simulink model "MultiVehicleModel"  (R2014a)
settings: Solver=ode1  StartTime=0.0  StopTime=inf  FixedStep=simPars.SampleTime  RelTol=1e-3
undefined symbols (not defined in the file or in its folder): DiscIntNeverNeededParam, Earth, Env, eul_0, FWFleet, GVFleet, m, RCFleet, s, WGS84
undefined symbols (not defined in the file): simPars
libraries: simulink x26, aerolibtransform2 x7, instrumentlib x6, Actuator_Lib x5, aerolib6dofsys x4, etargetslib x3, aerolibasang x3, aerolibconvert2 x2, aerolibutil x1, aerolibatmos2 x1, aerolibobsolete x1, aerolibgravity2 x1
(part 1 of 4)
settings Model: SimulationMode=accelerator  Creator=Paul Freeman  LastModifiedBy=Justyna
settings DataIOCC: LimitDataPoints=off  SignalLoggingSaveFormat=ModelDataLogs  SaveOutput=off  SignalLogging=off
settings OptimizationCC: ExpressionDepthLimit=2147483647  EfficientMapNaN2IntZero=off
settings DebuggingCC: UnderspecifiedInitializationDetection=Classic  MultiTaskDSMMsg=warning  MultiTaskCondExecSysMsg=none  FcnCallInpInsideContextMsg=UseLocalSettings  StateNameClashWarn=warning
settings HardwareCC: ProdLargestAtomicInteger=Long  ProdLargestAtomicFloat=Double  ProdIntDivRoundTo=Zero  ProdEndianess=BigEndian  ProdHWDeviceType=Freescale->32-bit PowerPC  TargetIntDivRoundTo=Zero  TargetEndianess=LittleEndian  TargetHWDeviceType=MATLAB Host  ProdEqTarget=off
settings SFSimCC: SimParseCustomCode=off
settings CodeAppCC: MaxIdLength=128
settings GRTTargetCC: CombineOutputUpdateFcns=off  GRTInterface=on

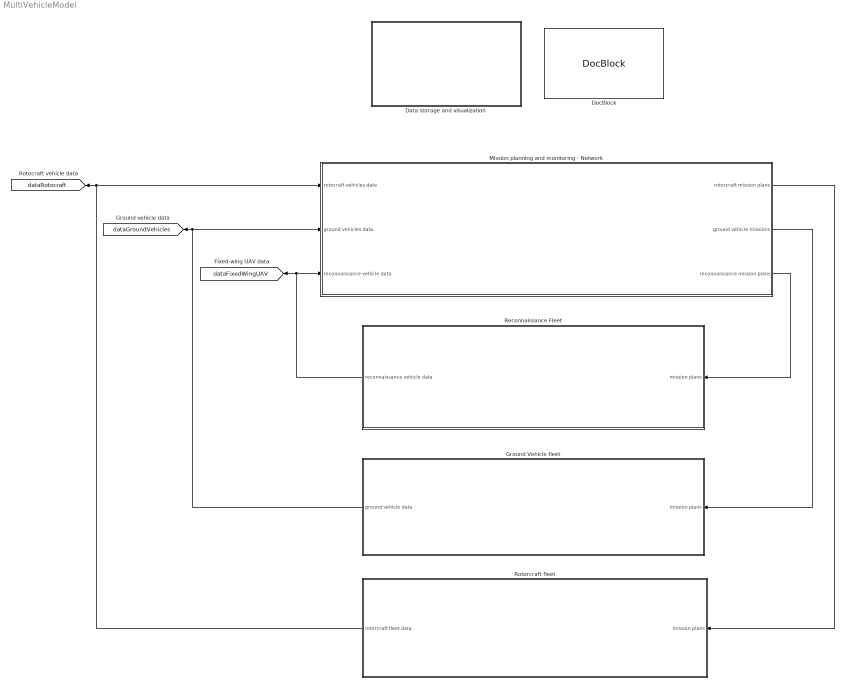
== system MultiVehicleModel ==
  Data storage and visualization : Subsystem
  DocBlock : simulink/Model-Wide Utilities/DocBlock  DocumentType=Text
      content=|
      | Type your documentation here
  Ground Vehicle fleet : Subsystem
  Mission planning and monitoring - Network : Subsystem  RequirementInfo={'other' 'specs1.mn' '@1.1.' 'true' 'specs' '' } %GIDa_c3d0c7d9_1841_4ce2_80a1_9c96a4f97ba6
  Reconnaissance Fleet : Subsystem
  Rotorcraft fleet : Subsystem
  tag scope: dataFixedWingUAV=global, dataGroundVehicles=global, dataRotocraft=global
  wires:
  Reconnaissance Fleet/1(reconnaissance vehicle data) -> [dataFixedWingUAV], Mission planning and monitoring - Network/3(reconnaissance vehicle data)
  Mission planning and monitoring - Network/3(reconnaissance mission plans) -> Reconnaissance Fleet/1(mission plans)
  Ground Vehicle fleet/1(ground vehicle data) -> [dataGroundVehicles], Mission planning and monitoring - Network/2(ground vehicles data)
  Rotorcraft fleet/1(rotorcraft fleet data) -> [dataRotocraft], Mission planning and monitoring - Network/1(rotocraft vehicles data)
  Mission planning and monitoring - Network/2(ground vehicle missions) -> Ground Vehicle fleet/1("mission plans ")
  Mission planning and monitoring - Network/1(rotorcraft mission plans) -> Rotorcraft fleet/1(mission plans)

== system MultiVehicleModel/Data storage and visualization ==
  To Workspace : ToWorkspace  VariableName=dataFixedWingUAV  SaveFormat=Structure With Time  SampleTime=-1
  To Workspace1 : ToWorkspace  VariableName=dataGroundVehicles  SaveFormat=Structure With Time  SampleTime=-1
  To Workspace2 : ToWorkspace  VariableName=dataRotorcraft  SaveFormat=Structure With Time  SampleTime=-1
  wires:
  [dataRotocraft] -> To Workspace2/1
  [dataGroundVehicles] -> To Workspace1/1
  [dataFixedWingUAV] -> To Workspace/1

== system MultiVehicleModel/Ground Vehicle fleet ==
  "mission plans " : Inport
  Bus Selector : BusSelector  OutputSignals=Ground vehicle fleet waypoints,Ground vehicle fleet functions
  Initial North-East-Down position : Constant  Value=GVFleet.IC.posNED(1:2,:)  VectorParams1D=off
  Model of ground vehicle fleet : Subsystem  TreatAsAtomicUnit=on  mask{AC=FWFleet.AC, Env=Env, SampleTime=simPars.SampleTime}
      mask prompts: AC "Aircraft properties"; Env "Environmental parameters"; SampleTime "Sample time (sec)"
  data inertial coordinates for debug. : ToWorkspace  VariableName=dataGVInertial  SaveFormat=Structure With Time  SampleTime=-1
  ground vehicle data : Outport
  wires:
  Model of ground vehicle fleet/1(output data) -> ground vehicle data/1
  Bus Selector/1 -> Model of ground vehicle fleet/1(air controller data)  "<Ground vehicle fleet waypoints>"
  Bus Selector/2 -> Model of ground vehicle fleet/2(AC fcn)  "<Ground vehicle fleet functions>"
  "mission plans "/1 -> Bus Selector/1
  Initial North-East-Down position/1 -> Model of ground vehicle fleet/3(Initial conditions)
  Model of ground vehicle fleet/2(output data inertial) -> data inertial coordinates for debug./1

== system MultiVehicleModel/Mission planning and monitoring - Network ==
  rotocraft vehicles data : Inport
  ground vehicles data : Inport  Port=2
  reconnaissance vehicle data : Inport  Port=3
  "Mission Plan Generation for fixed wing UAV fleet Runs on the server / cloud " : Subsystem
  Mission Plan Generation for ground vehicle fleet Runs on the server / cloud : Subsystem
  Mission Plan Generation for rotorcraft fleet Runs on the server / cloud : Subsystem
  rotorcraft mission plans : Outport
  ground vehicle missions : Outport  Port=2
  reconnaissance mission plans : Outport  Port=3
  wires:
  "Mission Plan Generation for fixed wing UAV fleet Runs on the server / cloud "/1(vehicle mission plans) -> reconnaissance mission plans/1  "vehicle mission plans"
  reconnaissance vehicle data/1 -> "Mission Plan Generation for fixed wing UAV fleet Runs on the server / cloud "/1(reconnaissance vehicle data)
  Mission Plan Generation for rotorcraft fleet Runs on the server / cloud/1(vehicle mission plans) -> rotorcraft mission plans/1
  ground vehicles data/1 -> Mission Plan Generation for ground vehicle fleet Runs on the server / cloud/1(ground vehicle data)
  rotocraft vehicles data/1 -> Mission Plan Generation for rotorcraft fleet Runs on the server / cloud/1(rotorcraft vehicle data)
  Mission Plan Generation for ground vehicle fleet Runs on the server / cloud/1(vehicle mission plans) -> ground vehicle missions/1

== system MultiVehicleModel/Reconnaissance Fleet ==
  mission plans : Inport
  Bus Selector : BusSelector  OutputSignals=Fixed-wing UAV fleet waypoints,Fixed-wing UAV fleet functions
  Initial North-East-Down position : Constant  Value=FWFleet.IC.posNED  VectorParams1D=off
  Initial heading : Constant  Value=FWFleet.IC.heading  VectorParams1D=off
  Matrix Concatenate : Concatenate  Mode=Multidimensional array
  UMN - Uninhabited Aerial Vehicle Fleet : Subsystem  TreatAsAtomicUnit=on  mask{AC=FWFleet.AC, Env=Env, SampleTime=simPars.SampleTime}
      mask prompts: AC "Aircraft properties"; Env "Environmental parameters"; SampleTime "Sample time (sec)"
  reconnaissance vehicle data : Outport
  wires:
  UMN - Uninhabited Aerial Vehicle Fleet/1(output data) -> reconnaissance vehicle data/1
  Bus Selector/1 -> UMN - Uninhabited Aerial Vehicle Fleet/1(mission plan)  "<Fixed-wing UAV fleet waypoints>"
  Bus Selector/2 -> UMN - Uninhabited Aerial Vehicle Fleet/2(Function)  "<Fixed-wing UAV fleet functions>"
  mission plans/1 -> Bus Selector/1
  Initial North-East-Down position/1 -> Matrix Concatenate/1
  Initial heading/1 -> Matrix Concatenate/2
  Matrix Concatenate/1 -> UMN - Uninhabited Aerial Vehicle Fleet/3(A/C initial conditions)

== system MultiVehicleModel/Rotorcraft fleet ==
  mission plans : Inport
  Bus Selector : BusSelector  OutputSignals="AR fleet waypoints,AR fleet heading and time,AR  fleet functions"
  Initial North-East-Down position : Constant  Value=RCFleet.IC.posNED  VectorParams1D=off
  Initial heading : Constant  Value=RCFleet.IC.heading  VectorParams1D=off
  Matrix Concatenate : Concatenate  Mode=Multidimensional array
  Multiple Rotorcraft : Subsystem  TreatAsAtomicUnit=on  mask{RCFleet=RCFleet}
      mask prompts: RCFleet "Rotorcraft fleet data structure"
  data inertial coordinates for debug. : ToWorkspace  VariableName=dataRotocraft2  SaveFormat=Structure With Time  SampleTime=-1
  rotorcraft fleet data : Outport
  wires:
  Multiple Rotorcraft/1(fleet states) -> rotorcraft fleet data/1
  Bus Selector/1 -> Multiple Rotorcraft/1(waypoints)  "<AR fleet waypoints>"
  Bus Selector/3 -> Multiple Rotorcraft/3(fleet functions)  "<AR  fleet functions>"
  mission plans/1 -> Bus Selector/1
  Multiple Rotorcraft/2(fleet inertial) -> data inertial coordinates for debug./1
  Bus Selector/2 -> Multiple Rotorcraft/2(heading and time references)  "<AR fleet heading and time>"
  Initial North-East-Down position/1 -> Matrix Concatenate/1
  Initial heading/1 -> Matrix Concatenate/2
  Matrix Concatenate/1 -> Multiple Rotorcraft/4(initial conditions)

== system MultiVehicleModel/Ground Vehicle fleet/Model of ground vehicle fleet ==
  air controller data : Inport  Partition=on  PartitionDimension=3  PartitionWidth=1
  AC fcn : Inport  Port=2  Partition=on  PartitionDimension=1  PartitionWidth=1
  Initial conditions : Inport  Port=3  Partition=on  PartitionDimension=2  PartitionWidth=1
  Bus Creator : BusCreator  Inputs=2
  Bus Selector1 : BusSelector  OutputSignals=Pned (m),psi (rad)
  Demux : Demux  Outputs=3
  Guidance algorithm : Subsystem
  Iteration over the UAV fleet : ForEach  DisableCoverage=on  IndexMode=One-based
  Mux1 : Mux
  Navigation : Subsystem  Description=|
      | This model produces the followng navigation data for the UAV flight:
      |                                                                     
      | * Geodetic Latitude                                                 
      | * Geodetic Longitude                                                
      | * Geodetic Altitude                                                 
      | * Altitude above Mean Sea Level                                     
      | * Gravitational acceleration vector
  Very simple car model : Subsystem
  data to send : Subsystem
  output data : Outport  ConcatenationDimension=1
  output data inertial : Outport  Port=2  ConcatenationDimension=1
  wires:
  air controller data/1 -> Guidance algorithm/2(waypoint data)
  AC fcn/1 -> Guidance algorithm/3(AC fcn)
  Very simple car model/1(position) -> Bus Creator/1, Navigation/1(X_e [m])  "Pned (m)"
  Very simple car model/2(heading (rad)) -> data to send/2(heading angle (rad)), Bus Creator/2  "psi (rad)"
  Bus Creator/1 -> Bus Selector1/1, Guidance algorithm/1(sensor data)
  Guidance algorithm/1(speed command (m/s)) -> Very simple car model/1(speed command (m/s))
  Guidance algorithm/2(heading command (rad)) -> Very simple car model/2(heading command (rad))
  Initial conditions/1 -> Very simple car model/3(initial inertial position X,Y (m))
  Mux1/1 -> output data inertial/1
  Bus Selector1/1 -> Demux/1  "<Pned (m)>"
  Bus Selector1/2 -> Mux1/4  "<psi (rad)>"
  Demux/3 -> Mux1/3
  Demux/2 -> Mux1/2
  Demux/1 -> Mux1/1
  Navigation/1(Nav) -> data to send/1(nav data)
  data to send/1(Data out) -> output data/1

== system MultiVehicleModel/Mission planning and monitoring - Network/Mission Plan Generation for fixed wing UAV fleet Runs on the server // cloud  ==
  reconnaissance vehicle data : Inport
  Bus Creator : BusCreator  Inputs=2
  Fixed wing vehicles' data to cloud : Subsystem
  Fleet Waypoint Reading from UDP : Subsystem
  vehicle mission plans : Outport
  wires:
  Bus Creator/1 -> vehicle mission plans/1
  Fleet Waypoint Reading from UDP/1(waypointsFleet) -> Bus Creator/1  "Fixed-wing UAV fleet waypoints"
  Fleet Waypoint Reading from UDP/2(fcnFleet) -> Bus Creator/2  "Fixed-wing UAV fleet functions"
  reconnaissance vehicle data/1 -> Fixed wing vehicles' data to cloud/1(UAV Fleet data)

== system MultiVehicleModel/Mission planning and monitoring - Network/Mission Plan Generation for ground vehicle fleet Runs on the server // cloud ==
  ground vehicle data : Inport
  Bus Creator : BusCreator  Inputs=2
  Fleet Waypoint Reading from UDP : Subsystem
  Ground vehicles' data to cloud : Subsystem
  vehicle mission plans : Outport
  wires:
  Bus Creator/1 -> vehicle mission plans/1
  Fleet Waypoint Reading from UDP/1(waypointsFleet) -> Bus Creator/1  "Ground vehicle fleet waypoints"
  Fleet Waypoint Reading from UDP/2(fcnFleet) -> Bus Creator/2  "Ground vehicle fleet functions"
  ground vehicle data/1 -> Ground vehicles' data to cloud/1(GV Fleet data)

== system MultiVehicleModel/Mission planning and monitoring - Network/Mission Plan Generation for rotorcraft fleet Runs on the server // cloud ==
  rotorcraft vehicle data : Inport
  Bus Creator : BusCreator  Inputs=3
  Fleet Waypoint Reading from UDP : Subsystem
  Rotorcraft vehicles' data to cloud : Subsystem
  vehicle mission plans : Outport
  wires:
  Bus Creator/1 -> vehicle mission plans/1
  Fleet Waypoint Reading from UDP/1(waypointsFleet) -> Bus Creator/1  "AR fleet waypoints"
  Fleet Waypoint Reading from UDP/3(fcnFleet) -> Bus Creator/3  "AR  fleet functions"
  rotorcraft vehicle data/1 -> Rotorcraft vehicles' data to cloud/1(UAV Fleet data)
  Fleet Waypoint Reading from UDP/2(Heading and Time) -> Bus Creator/2  "AR fleet heading and time"

== system MultiVehicleModel/Reconnaissance Fleet/UMN - Uninhabited Aerial Vehicle Fleet ==
  mission plan : Inport  Partition=on  PartitionDimension=3  PartitionWidth=1
  Function : Inport  Port=2  Partition=on  PartitionDimension=1  PartitionWidth=1
  A/C initial conditions : Inport  Port=3  Partition=on  PartitionDimension=2  PartitionWidth=1
  Actuators : Subsystem
  Control System : Subsystem  mask{control=AC.FC.control, IntegerTimeDelay=AC.FC.IntegerTimeDelay, TrimCondition=AC.TrimCondition, OperatingPoint=AC.OperatingPoint}
      mask prompts: control "Controller parameters"; IntegerTimeDelay "Integer Time Delay"; TrimCondition "Trim Condition"; OperatingPoint "Operating Point"
  Data packets to mission monitoring : Subsystem
  Guidance algorithm : Subsystem
  Iteration over the UAV fleet : ForEach  DisableCoverage=on  IndexMode=One-based
  Nonlinear UAV Model : Subsystem  mask{TrimCondition=AC.TrimCondition}
      mask prompts: TrimCondition "Trim Condition"
  Sensors : Subsystem
  output data : Outport  ConcatenationDimension=1
  wires:
  Sensors/1(Sensors) -> Guidance algorithm/1(sensor data), Control System/1(Sensors), Data packets to mission monitoring/1(" Vahicle data ")
  Nonlinear UAV Model/1(States) -> Sensors/1(States)
  Nonlinear UAV Model/2(EnvData) -> Sensors/2(EnvData)
  Control System/1(control_cmd) -> Actuators/1(cmds)
  Actuators/1(controls) -> Nonlinear UAV Model/1(Control Inputs)
  Guidance algorithm/1(ref_cmds) -> Control System/2(ref_cmds_in)
  mission plan/1 -> Guidance algorithm/2(waypoint data)
  A/C initial conditions/1 -> Nonlinear UAV Model/2(Initial conditions), [AC_IC]
  Function/1 -> Guidance algorithm/3(AC fcn)
  Data packets to mission monitoring/1(selected data out) -> output data/1
  [AC_IC] -> Guidance algorithm/4(initial inertial conditions)

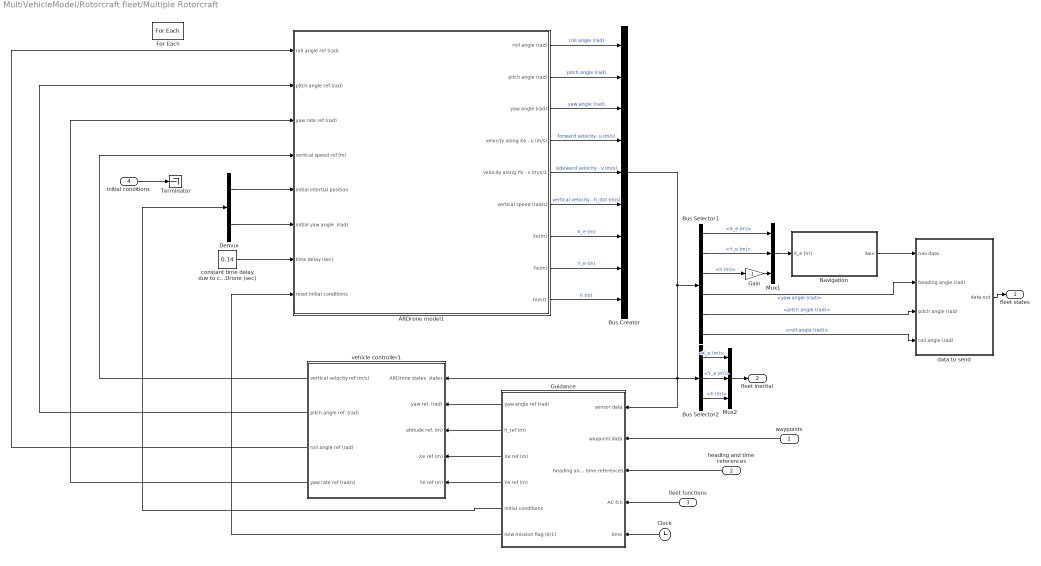
== system MultiVehicleModel/Rotorcraft fleet/Multiple Rotorcraft ==
  waypoints : Inport  Partition=on  PartitionDimension=3  PartitionWidth=1
  heading and time references : Inport  Port=2  Partition=on  PartitionDimension=3  PartitionWidth=1
  fleet functions : Inport  Port=3  Partition=on  PartitionDimension=1  PartitionWidth=1
  initial conditions : Inport  Port=4  Partition=on  PartitionDimension=2  PartitionWidth=1
  ARDrone model1 : Subsystem  mask{ARDrone=RCFleet.ARDrone}
      mask prompts: ARDrone "AR Drone parameters data structure"
  Bus Creator : BusCreator  Inputs=9
  Bus Selector1 : BusSelector  OutputSignals=X_e (m),Y_e (m),h (m),yaw angle (rad),pitch angle (rad),roll angle (rad)
  Bus Selector2 : BusSelector  OutputSignals=X_e (m),Y_e (m),h (m)
  Clock : Clock
  Demux : Demux  Outputs=[3 1]
  For Each : ForEach  DisableCoverage=on  IndexMode=One-based
  Gain : Gain  Gain=-1
  "Guidance " : Subsystem
  Mux1 : Mux  Inputs=3
  Mux2 : Mux  Inputs=3
  Navigation : Subsystem  Description=|
      | This model produces the followng navigation data for the UAV flight:
      |                                                                     
      | * Geodetic Latitude                                                 
      | * Geodetic Longitude                                                
      | * Geodetic Altitude                                                 
      | * Altitude above Mean Sea Level                                     
      | * Gravitational acceleration vector
  Terminator : Terminator
  constant time delay due to communications with ARDrone (sec) : Constant  Value=0.14
  data to send : Subsystem
  vehicle controller1 : Subsystem
  fleet states : Outport  ConcatenationDimension=1
  fleet inertial : Outport  Port=2  ConcatenationDimension=1
  wires:
  constant time delay due to communications with ARDrone (sec)/1 -> ARDrone model1/7(time delay (sec))
  Demux/2 -> ARDrone model1/6(initial yaw angle  (rad))
  ARDrone model1/1(roll angle (rad)) -> Bus Creator/1  "roll angle (rad)"
  ARDrone model1/2(pitch angle (rad)) -> Bus Creator/2  "pitch angle (rad)"
  ARDrone model1/3(yaw angle (rad)) -> Bus Creator/3  "yaw angle (rad)"
  ARDrone model1/4(velocity along Xb - u (m/s)) -> Bus Creator/4  "forward velocity- u (m/s)"
  ARDrone model1/5(velocity along Yb - v (m/s)1) -> Bus Creator/5  "sideward velocity - v (m/s)"
  ARDrone model1/6(vertical speed (rad/s)) -> Bus Creator/6  "vertical velocity - h_dot (m/s)"
  ARDrone model1/7(Xe(m)) -> Bus Creator/7  "X_e (m)"
  ARDrone model1/8(Ye(m)) -> Bus Creator/8  "Y_e (m)"
  ARDrone model1/9(h(m)1) -> Bus Creator/9  "h (m)"
  Bus Creator/1 -> "Guidance "/1(sensor data), Bus Selector2/1, vehicle controller1/1("ARDrone states  states "), Bus Selector1/1
  vehicle controller1/1(vertical velocity ref (m/s)) -> ARDrone model1/4(vertical speed ref (m))
  vehicle controller1/2(pitch angle ref. (rad)) -> ARDrone model1/2(pitch angle ref (rad))
  vehicle controller1/3(roll angle ref (rad)) -> ARDrone model1/1(roll angle ref (rad))
  vehicle controller1/4(yaw rate ref (rad/s)) -> ARDrone model1/3(yaw rate ref (rad))
  "Guidance "/3(Xe ref (m)) -> vehicle controller1/4(Xe ref (m))
  "Guidance "/4(Ye ref (m)) -> vehicle controller1/5(Ye ref (m))
  Clock/1 -> "Guidance "/5(time)
  "Guidance "/1(yaw angle ref (rad)) -> vehicle controller1/2(yaw ref. (rad))
  "Guidance "/2(h_ref (m)) -> vehicle controller1/3(altitude ref. (m))
  waypoints/1 -> "Guidance "/2(waypoint data)
  fleet functions/1 -> "Guidance "/4(AC fcn)
  Demux/1 -> ARDrone model1/5(initial intertial position)
  Bus Selector1/1 -> Mux1/1  "<X_e (m)>"
  Bus Selector1/3 -> Gain/1  "<h (m)>"
  Gain/1 -> Mux1/3
  Mux1/1 -> Navigation/1(X_e [m])
  Bus Selector1/2 -> Mux1/2  "<Y_e (m)>"
  Bus Selector2/1 -> Mux2/1  "<X_e (m)>"
  Bus Selector2/2 -> Mux2/2  "<Y_e (m)>"
  Bus Selector2/3 -> Mux2/3  "<h (m)>"
  Mux2/1 -> fleet inertial/1
  heading and time references/1 -> "Guidance "/3(heading and time references)
  Navigation/1(Nav) -> data to send/1(nav data)
  Bus Selector1/4 -> data to send/2(heading angle (rad))  "<yaw angle (rad)>"
  data to send/1(data out) -> fleet states/1
  "Guidance "/5(Initial conditions) -> Demux/1
  initial conditions/1 -> Terminator/1
  "Guidance "/6(new mission flag (0/1)) -> ARDrone model1/8(reset initial conditions)
  Bus Selector1/5 -> data to send/3(pitch angle (rad))  "<pitch angle (rad)>"
  Bus Selector1/6 -> data to send/4(roll angle (rad))  "<roll angle (rad)>"

== system MultiVehicleModel/Ground Vehicle fleet/Model of ground vehicle fleet/Guidance algorithm ==
  sensor data : Inport
  waypoint data : Inport  Port=2
  AC fcn : Inport  Port=3
  Bus Selector : BusSelector  OutputSignals=Pned (m)
  From geodetic to NED coordinate representation : Subsystem  TreatAsAtomicUnit=on
  Ground track angle computation based on waypoints : MATLAB Function  TreatAsAtomicUnit=on
  speed command (m/s) : Outport
  heading command (rad) : Outport  Port=2
  wires:
  AC fcn/1 -> Ground track angle computation based on waypoints/3(fcn)
  Ground track angle computation based on waypoints/1(vCmd) -> speed command (m/s)/1
  waypoint data/1 -> From geodetic to NED coordinate representation/1(geodetic [lat,lon,alt])
  From geodetic to NED coordinate representation/1("[N,E,D] (m)") -> Ground track angle computation based on waypoints/1(waypoint)
  sensor data/1 -> Bus Selector/1
  Bus Selector/1 -> Ground track angle computation based on waypoints/2(Pned)  "<Pned (m)>"
  Ground track angle computation based on waypoints/2(psiTarget) -> heading command (rad)/1

== system MultiVehicleModel/Ground Vehicle fleet/Model of ground vehicle fleet/Navigation ==
  X_e [m] : Inport
  Bus Creator1 : BusCreator  Inputs=6
  Demux : Demux  Outputs=2
  EGM-96 Geoid Model : Subsystem  mask(EGM-96 geoid undulation model){}
      mask help: Computes the MSL (mean sea level) altitude as a function of position.
      mask init:
      | load('egm96');
      mask Help:
      | The block computes the mean-sea-level altitude relative to the WGS-84 geoid.
      | <P><B>Inputs:</B>
      | <LI>Position = the 3x1 vector of aircraft location [Latitude Longitude Altitude], in [rad rad m]</LI>
      | </P>
      | <P><B>Output:</B>
      | <LI>MSLAlt = the mean-sea-level altitude, in m</LI>
      | </P>
  Flat Earth to LLA : aerolibtransform2/Flat Earth to LLA  units=Metric (MKS)  ptype=Earth (WGS84)  F=1/298.257223563  R=6378137  LL0=RCFleet.IC.geodetic(1:2)  psi=0
  Ground Detection : Subsystem  mask(Ground detection){}
      mask help: Computes altitude above ground and sets a flag if AGL is negative.
      mask Help:
      | The block computes the altitude above ground (AGL) and sets a flag if the AGL is negative (used for ground contact detection).
      | <P><B>Inputs:</B>
      | <LI>MSLAlt = the altitude measured from mean-sea-level, in meters</LI>
      | <LI>GndAlt = the altitude of the terrain (above MSL) at current location, in meters</LI>
      | </P>
      | <P><B>Output:</B>
      | <LI>AConGnd = the aircraft-on-ground flag (0 if aircraft above ground, 1 if aircraft on the ground)</LI>
      | <LI>AGLAlt = the altitude of the aircraft above ground</LI>
      | </P>
  Ground Height : Constant  Value=Env.GroundAlt
  Ground Height1 : Constant  Value=Env.GroundAlt
  Latitude Bound [-180,180] : Subsystem
  Longitude Bound 0-360 : Subsystem  mask(Longitude bound){}
      mask help: Bounds the longitude to [0, 2pi]. When 0 bound is exceeded the longitude wraps back to 2pi; when the 2pi bound is exceeded the longitude wraps back to 0.
  Mux : Mux  Inputs=3
  README : simulink/Model-Wide Utilities/DocBlock  DocumentType=Text
      content=|
      | Navigation
      |
      | This block is library link that contains the navigational model and
      | equations. Included are equations relating the flat Earth position to
      | latitude/longitude, a simplified 2D table lookup version of the EGM-96
      | Geoid model for computation of MSL/AGL altitudes, and computation of
      | flight path and ground track angles.
  Saturation : Saturate  UpperLimit=Inf  LowerLimit=0
  Nav : Outport
  wires:
  Ground Detection/2(AGLAlt) -> Bus Creator1/6  "Alt (Above Ground Level) [m]"
  Saturation/1 -> Mux/3, Bus Creator1/3  "Altitude [m]"
  Ground Detection/1(AConGnd) -> Bus Creator1/5  "AC on Ground"
  Ground Height1/1 -> Ground Detection/2(GndAlt)
  EGM-96 Geoid Model/1(MSLAlt) -> Bus Creator1/4, Ground Detection/1(MSLAlt)  "Alt (Above Mean Sea Level) [m]"
  Bus Creator1/1 -> Nav/1
  Ground Height/1 -> Flat Earth to LLA/2
  X_e [m]/1 -> Flat Earth to LLA/1
  Demux/2 -> Longitude Bound 0-360/1(In), Bus Creator1/2  "Geodetic Longitude [deg]"
  Demux/1 -> Bus Creator1/1, Latitude Bound [-180,180]/1(In)  "Geodetic Latitude [deg]"
  Flat Earth to LLA/2 -> Saturation/1  "Altitude [m]"
  Flat Earth to LLA/1 -> Demux/1
  Mux/1 -> EGM-96 Geoid Model/1(Position)
  Longitude Bound 0-360/1(Out) -> Mux/2
  Latitude Bound [-180,180]/1(Out) -> Mux/1

== system MultiVehicleModel/Ground Vehicle fleet/Model of ground vehicle fleet/Very simple car model ==
  speed command (m/s) : Inport
  heading command (rad) : Inport  Port=2
  initial inertial position X,Y (m) : Inport  Port=3
  "Car " : TransferFcn  Numerator=[30]  Denominator=[1 30]
  Car heading : TransferFcn  Denominator=[1]
  Integrator : Integrator  InitialConditionSource=external
  MATLAB Function : MATLAB Function  TreatAsAtomicUnit=on
  Mux : Mux  Inputs=3
  Mux1 : Mux  Inputs=2
  Saturation : Saturate  UpperLimit=30  LowerLimit=-30
  Z inertial pos (m) : Constant  Value=0
  Z inertial vel (m/s) : Constant  Value=0
  position : Outport
  heading (rad) : Outport  Port=2
  wires:
  heading command (rad)/1 -> Car heading/1
  speed command (m/s)/1 -> Saturation/1
  Saturation/1 -> "Car "/1
  "Car "/1 -> MATLAB Function/1(u)
  MATLAB Function/1(xNorthDot) -> Mux/1
  MATLAB Function/2(yEastDot) -> Mux/2
  Mux/1 -> Integrator/1
  Car heading/1 -> MATLAB Function/2(psi), heading (rad)/1
  Integrator/1 -> position/1
  Z inertial vel (m/s)/1 -> Mux/3
  initial inertial position X,Y (m)/1 -> Mux1/1
  Mux1/1 -> Integrator/2
  Z inertial pos (m)/1 -> Mux1/2

== system MultiVehicleModel/Ground Vehicle fleet/Model of ground vehicle fleet/data to send ==
  nav data : Inport
  heading angle (rad) : Inport  Port=2
  Bus Selector : BusSelector  OutputSignals=Geodetic Latitude [deg],Geodetic Longitude [deg],Altitude [m]
  Constant : Constant  Value=0
  Gain3 : Gain  Gain=180/pi
  Mux : Mux  Inputs=6
  Data out : Outport
  wires:
  Gain3/1 -> Mux/4
  heading angle (rad)/1 -> Gain3/1
  nav data/1 -> Bus Selector/1
  Bus Selector/1 -> Mux/1  "<Geodetic Latitude [deg]>"
  Bus Selector/2 -> Mux/2  "<Geodetic Longitude [deg]>"
  Bus Selector/3 -> Mux/3  "<Altitude [m]>"
  Mux/1 -> Data out/1
  Constant/1 -> Mux/5, Mux/6

== system MultiVehicleModel/Mission planning and monitoring - Network/Mission Plan Generation for fixed wing UAV fleet Runs on the server // cloud /Fixed wing vehicles' data to cloud ==
  UAV Fleet data : Inport
  Display : Display
  Rate Transition : RateTransition  OutPortSampleTimeOpt=Inherit  OutPortSampleTime=simPars.SampleTime
  UDP Send : instrumentlib/UDP Send  Host=127.0.0.1  Port=4043  LocalPort=-1  EnableBlockingMode=on  ByteOrder=LittleEndian
  wires:
  UAV Fleet data/1 -> Rate Transition/1
  Rate Transition/1 -> Display/1, UDP Send/1

== system MultiVehicleModel/Mission planning and monitoring - Network/Mission Plan Generation for fixed wing UAV fleet Runs on the server // cloud /Fleet Waypoint Reading from UDP ==
  Byte Unpack : etargetslib/Byte Unpack  dimensions={[3],[2],[300], [1]}  datatypes={'uint8', 'uint16', 'double','uint16'}  byteAlign=1
  Constant : Constant  Value=FWFleet.IC.geodetic
  "DataBase " : MATLAB Function  TreatAsAtomicUnit=on  mask{nAC=FWFleet.nFW, nWPs=FWFleet.nWPs}
      mask prompts: nAC "Number of vehicles in the fleet"; nWPs "Number of waypoints"
  Demux1 : Demux  Outputs=2
  UDP Receive : instrumentlib/UDP Receive  Host=0.0.0.0  Port=9080  LocalPort=9080  DataSize="[2409     1]"  EnableBlockingMode=off  Timeout=10  SampleTime=0.02  DataType=uint8  ByteOrder=BigEndian
  term0 : Terminator
  term1 : Terminator
  waypointsFleet : Outport
  fcnFleet : Outport  Port=2
  wires:
  "DataBase "/1(dataFleet) -> waypointsFleet/1
  Demux1/2 -> "DataBase "/2(functionID)
  UDP Receive/2 -> "DataBase "/4(status)
  Demux1/1 -> "DataBase "/1(uavID)
  Byte Unpack/3 -> "DataBase "/3(dataUAV)
  Byte Unpack/2 -> Demux1/1
  UDP Receive/1 -> Byte Unpack/1
  "DataBase "/2(fcnFleet) -> fcnFleet/1
  Byte Unpack/1 -> term0/1
  Byte Unpack/4 -> term1/1
  Constant/1 -> "DataBase "/5(LLA0)

== system MultiVehicleModel/Mission planning and monitoring - Network/Mission Plan Generation for ground vehicle fleet Runs on the server // cloud/Fleet Waypoint Reading from UDP ==
  Byte Unpack : etargetslib/Byte Unpack  dimensions={[3],[2],[300], [1]}  datatypes={'uint8', 'uint16', 'double','uint16'}  byteAlign=1
  Demux1 : Demux  Outputs=2
  GV initial geodetic position : Constant  Value=GVFleet.IC.geodetic
  UDP Receive : instrumentlib/UDP Receive  Host=0.0.0.0  Port=9040  LocalPort=9040  DataSize="[2409     1]"  EnableBlockingMode=off  Timeout=0.1  SampleTime=0.02  DataType=uint8  ByteOrder=BigEndian
  "data processing " : MATLAB Function  TreatAsAtomicUnit=on  mask{nAC=GVFleet.nGV}
      mask prompts: nAC "Number of vehicles in the fleet"
  term0 : Terminator
  term1 : Terminator
  waypointsFleet : Outport
  fcnFleet : Outport  Port=2
  wires:
  "data processing "/1(dataFleet) -> waypointsFleet/1
  Demux1/2 -> "data processing "/2(functionID)
  UDP Receive/2 -> "data processing "/4(status)
  Demux1/1 -> "data processing "/1(uavID)
  Byte Unpack/3 -> "data processing "/3(dataUAV)
  Byte Unpack/2 -> Demux1/1
  UDP Receive/1 -> Byte Unpack/1
  "data processing "/2(fcnFleet) -> fcnFleet/1
  Byte Unpack/1 -> term0/1
  Byte Unpack/4 -> term1/1
  GV initial geodetic position/1 -> "data processing "/5(LLA0)

== system MultiVehicleModel/Mission planning and monitoring - Network/Mission Plan Generation for ground vehicle fleet Runs on the server // cloud/Ground vehicles' data to cloud ==
  GV Fleet data : Inport
  Display : Display
      settings: Format=long_e
  Rate Transition : RateTransition  OutPortSampleTimeOpt=Inherit  OutPortSampleTime=simPars.SampleTime
  To Optimization  module : instrumentlib/UDP Send  Host=127.0.0.1  Port=4042  LocalPort=-1  EnableBlockingMode=on  ByteOrder=LittleEndian
  wires:
  GV Fleet data/1 -> Rate Transition/1
  Rate Transition/1 -> Display/1, To Optimization  module/1

== system MultiVehicleModel/Mission planning and monitoring - Network/Mission Plan Generation for rotorcraft fleet Runs on the server // cloud/Fleet Waypoint Reading from UDP ==
  Byte Unpack : etargetslib/Byte Unpack  dimensions={[3],[2],[500], [1]}  datatypes={'uint8', 'uint16', 'double','uint16'}  byteAlign=1
  Constant : Constant  Value=RCFleet.IC.geodetic
  "DataBase " : MATLAB Function  TreatAsAtomicUnit=on  mask{nAC=RCFleet.nRC}
      mask prompts: nAC "Number of vehicles in the fleet"
  Demux1 : Demux  Outputs=2
  UDP Receive : instrumentlib/UDP Receive  Host=0.0.0.0  Port=9020  LocalPort=9020  DataSize="[4009     1]"  EnableBlockingMode=off  Timeout=10  SampleTime=0.02  DataType=uint8  ByteOrder=BigEndian
  term0 : Terminator
  term1 : Terminator
  waypointsFleet : Outport
  Heading and Time : Outport  Port=2
  fcnFleet : Outport  Port=3
  wires:
  "DataBase "/1(dataWP) -> waypointsFleet/1
  Demux1/2 -> "DataBase "/2(functionID)
  UDP Receive/2 -> "DataBase "/4(status)
  Demux1/1 -> "DataBase "/1(uavID)
  Byte Unpack/3 -> "DataBase "/3(dataUAV)
  Byte Unpack/2 -> Demux1/1
  UDP Receive/1 -> Byte Unpack/1
  "DataBase "/3(fcnFleet) -> fcnFleet/1
  Byte Unpack/1 -> term0/1
  Byte Unpack/4 -> term1/1
  "DataBase "/2(dataHT) -> Heading and Time/1
  Constant/1 -> "DataBase "/5(LLA0)

== system MultiVehicleModel/Mission planning and monitoring - Network/Mission Plan Generation for rotorcraft fleet Runs on the server // cloud/Rotorcraft vehicles' data to cloud ==
  UAV Fleet data : Inport
  Display : Display
      settings: Format=long_e
  Rate Transition : RateTransition  OutPortSampleTimeOpt=Inherit  OutPortSampleTime=simPars.SampleTime
  Scope : Scope
      settings: YMin=-130  YMax=50
  UDP Send : instrumentlib/UDP Send  Host=127.0.0.1  Port=4044  LocalPort=-1  EnableBlockingMode=on  ByteOrder=LittleEndian
  wires:
  UAV Fleet data/1 -> Rate Transition/1
  Rate Transition/1 -> Scope/1, Display/1, UDP Send/1

== system MultiVehicleModel/Reconnaissance Fleet/UMN - Uninhabited Aerial Vehicle Fleet/Actuators ==
  cmds : Inport
  Bus Creator : BusCreator  Inputs=7
  Demux : Demux  Outputs=7
  Elevator Servo : Subsystem  mask(Rate and Position Limited Servo){freq=AC.Actuator.elevator.BW, RL=AC.Actuator.elevator.RateLim, POS_hi=AC.Actuator.elevator.PosLim, POS_lo=AC.Actuator.elevator.NegLim}
      mask prompts: freq "Bandwidth, Hz"; RL "Rate Limit:"; POS_hi "Position Limit High:"; POS_lo "Position Limit Low:"
      mask help: First order transfer function: w/(s+w), with rate and position limits.
      mask Help:
      | This block models a first order servo with the initial condition
      | on the integrator set to the steady state value for constant input.
      | The servo is rate and position limited and those values are set
      | in the block parameters.
      mask Display:
      | text(.48,.55,sprintf('%3.1f Hz\nBW',freq),'horizontalAlignment','center');
      | 
      | text(0.18,0.45,sprintf('|d/dt|\n<%0.1f',RL),'horizontalAlignment','center');
      | 
      | text(0.88,0.85,num2str(POS_hi),'horizontalAlignment', 'center');
      | text(0.88,0.2,num2str(POS_lo),'horizontalAlignment', 'center');
      | text(0.73,0.5,'P\nL');
      | 
      | 
      | plot([0.83 0.87 0.93 0.97],[0.4 0.4 0.6 0.6]);
      | plot([0.81 0.99],[0.5 0.5]);
      | plot([0.9 0.9],[0.3 0.7]);
      | plot([0.81 0.99 0.99 0.81 0.81],[0.3 0.3 0.7 0.7 0.3]);
  Left Aileron Servo : Subsystem  mask(Rate and Position Limited Servo){freq=AC.Actuator.l_aileron.BW, RL=AC.Actuator.l_aileron.RateLim, POS_hi=AC.Actuator.l_aileron.PosLim, POS_lo=AC.Actuator.l_aileron.NegLim}
      mask prompts: freq "Bandwidth, Hz"; RL "Rate Limit:"; POS_hi "Position Limit High:"; POS_lo "Position Limit Low:"
      mask help: First order transfer function: w/(s+w), with rate and position limits.
      mask Help:
      | This block models a first order servo with the initial condition
      | on the integrator set to the steady state value for constant input.
      | The servo is rate and position limited and those values are set
      | in the block parameters.
      mask Display:
      | text(.48,.55,sprintf('%3.1f Hz\nBW',freq),'horizontalAlignment','center');
      | 
      | text(0.18,0.45,sprintf('|d/dt|\n<%0.1f',RL),'horizontalAlignment','center');
      | 
      | text(0.88,0.85,num2str(POS_hi),'horizontalAlignment', 'center');
      | text(0.88,0.2,num2str(POS_lo),'horizontalAlignment', 'center');
      | text(0.73,0.5,'P\nL');
      | 
      | 
      | plot([0.83 0.87 0.93 0.97],[0.4 0.4 0.6 0.6]);
      | plot([0.81 0.99],[0.5 0.5]);
      | plot([0.9 0.9],[0.3 0.7]);
      | plot([0.81 0.99 0.99 0.81 0.81],[0.3 0.3 0.7 0.7 0.3]);
  Left Flap Servo : Subsystem  mask(Rate and Position Limited Servo){freq=AC.Actuator.l_flap.BW, RL=AC.Actuator.l_flap.RateLim, POS_hi=AC.Actuator.l_flap.PosLim, POS_lo=AC.Actuator.l_flap.NegLim}
      mask prompts: freq "Bandwidth, Hz"; RL "Rate Limit:"; POS_hi "Position Limit High:"; POS_lo "Position Limit Low:"
      mask help: First order transfer function: w/(s+w), with rate and position limits.
      mask Help:
      | This block models a first order servo with the initial condition
      | on the integrator set to the steady state value for constant input.
      | The servo is rate and position limited and those values are set
      | in the block parameters.
      mask Display:
      | text(.48,.55,sprintf('%3.1f Hz\nBW',freq),'horizontalAlignment','center');
      | 
      | text(0.18,0.45,sprintf('|d/dt|\n<%0.1f',RL),'horizontalAlignment','center');
      | 
      | text(0.88,0.85,num2str(POS_hi),'horizontalAlignment', 'center');
      | text(0.88,0.2,num2str(POS_lo),'horizontalAlignment', 'center');
      | text(0.73,0.5,'P\nL');
      | 
      | 
      | plot([0.83 0.87 0.93 0.97],[0.4 0.4 0.6 0.6]);
      | plot([0.81 0.99],[0.5 0.5]);
      | plot([0.9 0.9],[0.3 0.7]);
      | plot([0.81 0.99 0.99 0.81 0.81],[0.3 0.3 0.7 0.7 0.3]);
  README : simulink/Model-Wide Utilities/DocBlock  DocumentType=Text
      content=|
      | Actuators
      |
      | This block implements first order, rate and position limited actuator
      | models for the aileron, elevator, rudder and flap channels. The throttle
      | does not have a servo, but is position limited.
      |
      | Parameters for these models are contained in the aircraft configuration
      | data structure variable, "AC". Specfically,
      |
      | >> AC.Actuator
      |
      | ans =
      |
      |      elevator: [1x1 struct]
      |     l_aileron: [1x1 struct]
      |     r_aileron: [1x1 struct]
      |        rudder: [1x1 struct]
      |        l_flap: [1x1 struct]
      |        r_flap: [1x1 struct]
      |      throttle: [1x1 struct]
      |
      | Control Inputs Sign Convention
      | Elevator: +TED
      | Rudder: +TEL
      | Ailerons: +TED, da = (da_R-da_L)/2
      | Flaps: +TED
      | Throttle: always positive
  Right Aileron Servo : Subsystem  mask(Rate and Position Limited Servo){freq=AC.Actuator.r_aileron.BW, RL=AC.Actuator.r_aileron.RateLim, POS_hi=AC.Actuator.r_aileron.PosLim, POS_lo=AC.Actuator.r_aileron.NegLim}
      mask prompts: freq "Bandwidth, Hz"; RL "Rate Limit:"; POS_hi "Position Limit High:"; POS_lo "Position Limit Low:"
      mask help: First order transfer function: w/(s+w), with rate and position limits.
      mask Help:
      | This block models a first order servo with the initial condition
      | on the integrator set to the steady state value for constant input.
      | The servo is rate and position limited and those values are set
      | in the block parameters.
      mask Display:
      | text(.48,.55,sprintf('%3.1f Hz\nBW',freq),'horizontalAlignment','center');
      | 
      | text(0.18,0.45,sprintf('|d/dt|\n<%0.1f',RL),'horizontalAlignment','center');
      | 
      | text(0.88,0.85,num2str(POS_hi),'horizontalAlignment', 'center');
      | text(0.88,0.2,num2str(POS_lo),'horizontalAlignment', 'center');
      | text(0.73,0.5,'P\nL');
      | 
      | 
      | plot([0.83 0.87 0.93 0.97],[0.4 0.4 0.6 0.6]);
      | plot([0.81 0.99],[0.5 0.5]);
      | plot([0.9 0.9],[0.3 0.7]);
      | plot([0.81 0.99 0.99 0.81 0.81],[0.3 0.3 0.7 0.7 0.3]);
  Right Flap Servo : Subsystem  mask(Rate and Position Limited Servo){freq=AC.Actuator.l_flap.BW, RL=AC.Actuator.l_flap.RateLim, POS_hi=AC.Actuator.l_flap.PosLim, POS_lo=AC.Actuator.l_flap.NegLim}
      mask prompts: freq "Bandwidth, Hz"; RL "Rate Limit:"; POS_hi "Position Limit High:"; POS_lo "Position Limit Low:"
      mask help: First order transfer function: w/(s+w), with rate and position limits.
      mask Help:
      | This block models a first order servo with the initial condition
      | on the integrator set to the steady state value for constant input.
      | The servo is rate and position limited and those values are set
      | in the block parameters.
      mask Display:
      | text(.48,.55,sprintf('%3.1f Hz\nBW',freq),'horizontalAlignment','center');
      | 
      | text(0.18,0.45,sprintf('|d/dt|\n<%0.1f',RL),'horizontalAlignment','center');
      | 
      | text(0.88,0.85,num2str(POS_hi),'horizontalAlignment', 'center');
      | text(0.88,0.2,num2str(POS_lo),'horizontalAlignment', 'center');
      | text(0.73,0.5,'P\nL');
      | 
      | 
      | plot([0.83 0.87 0.93 0.97],[0.4 0.4 0.6 0.6]);
      | plot([0.81 0.99],[0.5 0.5]);
      | plot([0.9 0.9],[0.3 0.7]);
      | plot([0.81 0.99 0.99 0.81 0.81],[0.3 0.3 0.7 0.7 0.3]);
  Rudder Servo : Subsystem  mask(Rate and Position Limited Servo){freq=AC.Actuator.rudder.BW, RL=AC.Actuator.rudder.RateLim, POS_hi=AC.Actuator.rudder.PosLim, POS_lo=AC.Actuator.rudder.NegLim}
      mask prompts: freq "Bandwidth, Hz"; RL "Rate Limit:"; POS_hi "Position Limit High:"; POS_lo "Position Limit Low:"
      mask help: First order transfer function: w/(s+w), with rate and position limits.
      mask Help:
      | This block models a first order servo with the initial condition
      | on the integrator set to the steady state value for constant input.
      | The servo is rate and position limited and those values are set
      | in the block parameters.
      mask Display:
      | text(.48,.55,sprintf('%3.1f Hz\nBW',freq),'horizontalAlignment','center');
      | 
      | text(0.18,0.45,sprintf('|d/dt|\n<%0.1f',RL),'horizontalAlignment','center');
      | 
      | text(0.88,0.85,num2str(POS_hi),'horizontalAlignment', 'center');
      | text(0.88,0.2,num2str(POS_lo),'horizontalAlignment', 'center');
      | text(0.73,0.5,'P\nL');
      | 
      | 
      | plot([0.83 0.87 0.93 0.97],[0.4 0.4 0.6 0.6]);
      | plot([0.81 0.99],[0.5 0.5]);
      | plot([0.9 0.9],[0.3 0.7]);
      | plot([0.81 0.99 0.99 0.81 0.81],[0.3 0.3 0.7 0.7 0.3]);
  throttle limits : Saturate  UpperLimit=AC.Actuator.throttle.PosLim  LowerLimit=AC.Actuator.throttle.NegLim
  controls : Outport
  wires:
  Bus Creator/1 -> controls/1
  cmds/1 -> Demux/1
  Demux/1 -> throttle limits/1
  throttle limits/1 -> Bus Creator/1  "throttle [nd]"
  Demux/2 -> Elevator Servo/1(In)
  Elevator Servo/1(Out) -> Bus Creator/2  "elevator [rad]"
  Demux/3 -> Rudder Servo/1(In)
  Rudder Servo/1(Out) -> Bus Creator/3  "rudder [rad]"
  Demux/4 -> Left Aileron Servo/1(In)
  Left Aileron Servo/1(Out) -> Bus Creator/4  "l_aileron [rad]"
  Demux/6 -> Left Flap Servo/1(In)
  Left Flap Servo/1(Out) -> Bus Creator/6  "l_flap [rad]"
  Right Aileron Servo/1(Out) -> Bus Creator/5  "r_aileron [rad]"
  Right Flap Servo/1(Out) -> Bus Creator/7  "r_flap [rad]"
  Demux/7 -> Right Flap Servo/1(In)
  Demux/5 -> Right Aileron Servo/1(In)

== system MultiVehicleModel/Reconnaissance Fleet/UMN - Uninhabited Aerial Vehicle Fleet/Control System ==
  note: See "Software\Documentation\UAV_controllaw_ICD.pdf" for
      | details on the input/output signals.
  Sensors : Inport
  ref_cmds_in : Inport  Port=2
  Bus Creator : BusCreator  Inputs=7
  Bus Selector1 : BusSelector  OutputSignals=phi [rad],theta [rad],psi [rad],p [rad/s],q [rad/s],r [rad/s],Ax [m/s^2],Ay [m/s^2],Az [m/s^2],h [m],V_s [m/s],alpha [rad],beta [rad],Geodetic Latitude [rad],Geodetic Longitude [rad],Altitude [m],Xdot [m/s],Ydot [m/s],Zdot [m/s]  OutputAsBus=on
  "Control_Algorithm " : Subsystem
  Demux : Demux  Outputs=7
  Integer Delay : Delay  DelayLength=IntegerTimeDelay  InitialCondition=repmat([TrimCondition.AttitudeIni;TrimCondition.RatesIni;TrimCondition.AccelsIni;OperatingPoint.op_report.Outputs(4).y;TrimCondition.WindAxesIni;TrimCondition.LLIni;0; zeros(3,1)],[1,IntegerTimeDelay])  InputProcessing=Inherited
  README : simulink/Model-Wide Utilities/DocBlock  DocumentType=Text
      content=|
      | Control Law Block
      |
      | This block uses Model Referencing to allow the user to easily switch out
      | control law implementations. An example usage would be first a user develops
      | a control law using simulink blocks. This controller is referred to as the
      | "simulink controller" and would be selected by setting the variable
      | "controller_mode" to 2. Once the development is completed, the user then
      | implements the Simulink controller into C-code suitable for integration
      | with the UAV software. This controller is referred to as the "flight code"
      | and would be selected by setting "controller_mode" to 1.
      |
      | This is done using the Simulink.Variant object. See the documentation for
      | more detail. The user can specify any number of variants for the Control
      | Software block; edit the ModelReferenceParameters by right-clicking this
      | block to set which Simulink model is reference for each Variant object.
      | Note that these objects must be present in the base workspace. It
      | is strongly recommended that you use the "simulink_controller.mdl" file as
      | a starting place and "Save As" to a different file name.
      |
      | In summary, to switch the Control Software, modify the "contoller_mode"
      | variable:
      | 1 = flight code controller (C implementation)
      | 2 = simulink controller (empty simulink model)
      |
      |
      | See "Software\Documentation\UAV_controllaw_ICD.pdf" for details on the
      | input/output signals.
      |
      | The control_cmd signal must have the following order:
      | throttle
      | elevator
      | rudder
      | l_aileron
      | r_aileron
      | l_flap
      | r_flap
      |
      | Control Inputs Sign Convention
      | TED = Trailing Edge Down
      | TEL = Trailing Edge Left
      | ------------------------
      | Elevator: +TED
      | Rudder: +TEL
      | Aileron: +TED, da = (da_R-da_L)/2
      | Throttle: always positive
      | Flap: +TED
      |
      |
      | The refrence command signal must have the following order:
      | 1. phi_cmd
      | 2. theta_cmd
      | 3. psi_cmd
      | 4. p_cmd
      | 5. q_cmd
      | 6. r_cmd
      | 7. V_s_cmd
      | 8. h_cmd
      | 9. gndtrk_cmd
      | 10. aoa_cmd
      | 11. aos_cmd
      | 12. gamma_cmd
      | Note the trimmed value of pitch angle theta is included in the reference
      | command. Use the Doublet Generator block (or other signal generating block)
      | to input reference commands to the Control Software.
  Terminator : Terminator
  "Trim setting " : Actuator_Lib/Trim setting 
  control_cmd : Outport
  wires:
  "Control_Algorithm "/1(control_cmd1) -> "Trim setting "/1
  Sensors/1 -> Bus Selector1/1
  ref_cmds_in/1 -> "Control_Algorithm "/2(ref_cmds)
  Bus Creator/1 -> control_cmd/1
  Demux/1 -> Bus Creator/1  "throttle [nd]"
  Demux/2 -> Bus Creator/2  "elevator [rad]"
  Demux/3 -> Bus Creator/3  "rudder [rad]"
  Demux/4 -> Bus Creator/4  "l_aileron [rad]"
  Demux/5 -> Bus Creator/5  "r_aileron [rad]"
  Demux/6 -> Bus Creator/6  "l_flap [rad]"
  Demux/7 -> Bus Creator/7  "r_flap [rad]"
  Integer Delay/1 -> "Control_Algorithm "/1(feedback)
  Bus Selector1/1 -> Integer Delay/1
  "Trim setting "/1 -> Demux/1
  "Control_Algorithm "/2(ref_cmds_out) -> Terminator/1

== system MultiVehicleModel/Reconnaissance Fleet/UMN - Uninhabited Aerial Vehicle Fleet/Data packets to mission monitoring ==
  " Vahicle data " : Inport
  Bus Selector3 : BusSelector  OutputSignals=Geodetic Latitude [rad],Geodetic Longitude [rad],Altitude [m],psi [rad],theta [rad],phi [rad]
  Gain : Gain  Gain=180/pi
  Gain1 : Gain  Gain=180/pi
  Gain2 : Gain  Gain=-180/pi
  Gain3 : Gain  Gain=180/pi
  Gain4 : Gain  Gain=-180/pi
  Mux : Mux  Inputs=6
  selected data out : Outport
  wires:
  Gain1/1 -> Mux/2
  Gain3/1 -> Mux/4
  " Vahicle data "/1 -> Bus Selector3/1
  Gain/1 -> Mux/1
  Bus Selector3/1 -> Gain/1  "<Geodetic Latitude [rad]>"
  Mux/1 -> selected data out/1
  Bus Selector3/2 -> Gain1/1  "<Geodetic Longitude [rad]>"
  Bus Selector3/3 -> Mux/3  "<Altitude [m]>"
  Bus Selector3/4 -> Gain3/1  "<psi [rad]>"
  Bus Selector3/5 -> Gain2/1  "<theta [rad]>"
  Bus Selector3/6 -> Gain4/1  "<phi [rad]>"
  Gain2/1 -> Mux/5
  Gain4/1 -> Mux/6

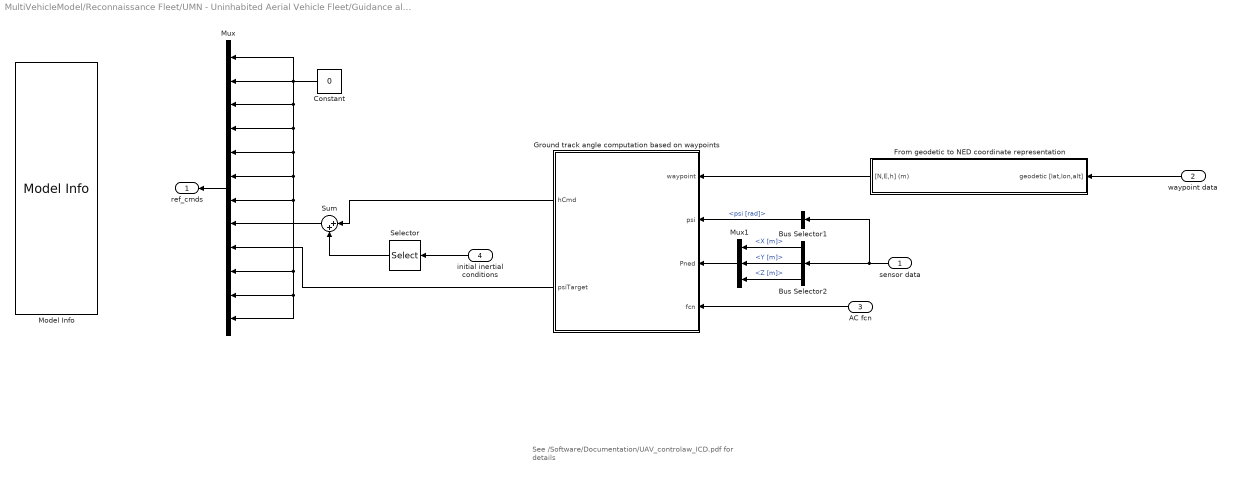
== system MultiVehicleModel/Reconnaissance Fleet/UMN - Uninhabited Aerial Vehicle Fleet/Guidance algorithm ==
  note: See /Software/Documentation/UAV_controlaw_ICD.pdf
      | for details
  sensor data : Inport
  waypoint data : Inport  Port=2
  AC fcn : Inport  Port=3
  initial inertial conditions : Inport  Port=4
  Bus Selector1 : BusSelector  OutputSignals=psi [rad]
  Bus Selector2 : BusSelector  OutputSignals=X_e [m].X [m],X_e [m].Y [m],X_e [m].Z [m]
  Constant : Constant  Value=0
  From geodetic to NED coordinate representation : Subsystem  TreatAsAtomicUnit=on
  Ground track angle computation based on waypoints : MATLAB Function  TreatAsAtomicUnit=on
  Model Info : simulink/Model-Wide Utilities/Model Info  InitialBlockCM=None  Frame=on  DisplayStringWithTags=|  HorizontalTextAlignment=Center  LeftAlignmentValue=0.5  SourceBlockDiagram=MultiVehicleModel  TagMaxNumber=20
      | Ref Cmd Port Info
      | 
      | 1. phi_cmd
      | 2. theta_cmd
      | 3. psi_cmd
      | 4. p_cmd
      | 5. q_cmd
      | 6. r_cmd
      | 7. V_s_cmd
      | 8. h_cmd
      | 9. gndtrk_cmd
      | 10. aoa_cmd
      | 11. aos_cmd
      | 12. gamma_cmd
  Mux : Mux  Inputs=12
  Mux1 : Mux  Inputs=3
  Selector : Selector  InputPortWidth=4  Indices=[3]
  Sum : Sum  Inputs=|++
  ref_cmds : Outport
  wires:
  Mux/1 -> ref_cmds/1
  Bus Selector2/1 -> Mux1/1  "<X [m]>"
  Bus Selector2/2 -> Mux1/2  "<Y [m]>"
  Bus Selector2/3 -> Mux1/3  "<Z [m]>"
  sensor data/1 -> Bus Selector1/1, Bus Selector2/1
  Bus Selector1/1 -> Ground track angle computation based on waypoints/2(psi)  "<psi [rad]>"
  Mux1/1 -> Ground track angle computation based on waypoints/3(Pned)
  Ground track angle computation based on waypoints/2(psiTarget) -> Mux/9
  Constant/1 -> Mux/3, Mux/4, Mux/5, Mux/6, Mux/7, Mux/10, Mux/11, Mux/12, Mux/1, Mux/2
  AC fcn/1 -> Ground track angle computation based on waypoints/4(fcn)
  Sum/1 -> Mux/8
  Ground track angle computation based on waypoints/1(hCmd) -> Sum/1
  waypoint data/1 -> From geodetic to NED coordinate representation/1(geodetic [lat,lon,alt])
  From geodetic to NED coordinate representation/1("[N,E,h] (m)") -> Ground track angle computation based on waypoints/1(waypoint)
  initial inertial conditions/1 -> Selector/1
  Selector/1 -> Sum/2

== system MultiVehicleModel/Reconnaissance Fleet/UMN - Uninhabited Aerial Vehicle Fleet/Nonlinear UAV Model ==
  Control Inputs : Inport
  Initial conditions : Inport  Port=2
  6DoF EOM : Subsystem  mask(6DoF EoM (Body Axis)){units=Metric (MKS), mtype=Fixed, rep=Euler Angles, xme_0=TrimCondition.InertialIni, Vm_0=TrimCondition.VelocitiesIni, pm_0=TrimCondition.RatesIni, mass_0=AC.Mass, mass_e=0.5, mass_f=2.0, inertia=AC.Inertia.Matrix, inertia_e=eye(3), inertia_f=2*eye(3), k_quat=1.0}
      mask prompts: mtype "Mass type:"; rep "Representation:"; xme_0 "Initial position in inertial axes [Xe,Ye,Ze]:"; Vm_0 "Initial velocity in body axes [U,v,w]:"; pm_0 "Initial body rotation rates [p,q,r]:"; mass_0 "Initial mass:"; mass_e "Empty mass:"; mass_f "Full mass:"; inertia_e "Empty inertia matrix:"; inertia_f "Full inertia matrix:"; k_quat "Gain for quaternion normalization:"
      mask help:
      | Integrate the six-degrees-of-freedom equations of motion in body axis.
      |
      | This block has been modified from the original Aerospace Blockset
      | implementation. The inertial position vector (Xe) is no longer computed.
      | The original block did not have a way to add steady state winds to the
      | inertial velocities (Ve) prior to integrating to get Xe. Therefore, this
      | step is performed in the Auxiliary Equations block.
      mask Help: eval('asbhelp(''sixdof_euler_angles'')');
      mask TypeOptions units: Metric (MKS) | English (Velocity in ft/s) | English (Velocity in kts)
      mask TypeOptions mtype: Fixed | Simple Variable | Custom Variable
      mask Callback mtype: aeroicon('aeroblk6dofbody');
      mask TypeOptions rep: Euler Angles | Quaternion
      mask Callback rep: aeroicon('aeroblk6dofbody');
  Auxiliary Equations : Subsystem
  Environment : Subsystem
  Forces and Moments : Subsystem
  Initial conditions1 : InportShadow  Port=2
  "Packaging initial Euler angles " : Subsystem
  README : simulink/Model-Wide Utilities/DocBlock  DocumentType=Text
      content=|
      | Nonlinear UAV Model
      |
      | This block implements the nonlinear UAV dynamics model. Beginning on the
      | left, the Forces and Moments block models all of the relevant external
      | forces and moments acting on the aircraft.
      |
      | The 6DoF EOM block implements the six degree of freedom, fixed mass,
      | flat, non-rotating Earth, rigid body equations of motion. This block has
      | been modified from the original Aerospace Blockset implementation. The
      | inertial position vector (Xe) is no longer computed. The original block
      | did not have a way to add steady state winds to the inertial velocities
      | (Ve) prior to integrating to get Xe. Therefore, this step is performed in
      | the Auxiliary Equations block.
      |
      | The Auxiliary Equations computes other relevant variables (such as angle
      | of attack, indicated airspeed, etc) from state data. In this block are
      | the Navigation equations.
      |
      | Finally, the Environment block has Aerospace Blockset models for Earth's
      | atmosphere, gravity, and magnetic fields. Winds are modeled in two
      | portions: steady and unsteady. The steady portion is defined by a speed
      | and direction, and is horizontal only. The unsteady portion is made up of
      | a wind shear model and a turbulence model.
  States : Outport
  EnvData : Outport  Port=2
  wires:
  6DoF EOM/6(Ab) -> Auxiliary Equations/6(A_b)
  6DoF EOM/5(pdot,qdot,rdot) -> Auxiliary Equations/5(AngAccel)
  6DoF EOM/4(p,q,r) -> Auxiliary Equations/4(AngVel)
  6DoF EOM/3(Vb) -> Auxiliary Equations/3(V_b)
  6DoF EOM/2(DCM) -> Auxiliary Equations/2(DCM)
  6DoF EOM/1(Euler) -> Auxiliary Equations/1(Euler)
  Control Inputs/1 -> Forces and Moments/1(Control Inputs)
  Forces and Moments/1(Total Force) -> 6DoF EOM/1(Forces)
  Forces and Moments/2(Total Moment) -> 6DoF EOM/2(Moments)
  Auxiliary Equations/1(States) -> States/1, Forces and Moments/2(States), Environment/1(States)
  Forces and Moments/3(nonGravForces) -> Auxiliary Equations/7(NonGravForces)
  Environment/1(EnvData) -> Forces and Moments/3(EnvData), Auxiliary Equations/8(EnvData), EnvData/1
  Initial conditions/1 -> Auxiliary Equations/9(Initial conditions)
  Initial conditions1/1 -> "Packaging initial Euler angles "/1(Position and heading)
  "Packaging initial Euler angles "/1(Initial Euler angles) -> 6DoF EOM/3(Euler ini. (rad))
